simulink model "LQI_control"  (R2020a)
settings: Solver=ode4  StartTime=0.0  StopTime=t  FixedStep=0.01  RelTol=1e-3
values from neighbouring files (symbols this model uses):
  A = [-0.0226 -36.6 -18.9 -32.1 ;            0 -1.9  0.983     0;       0.0123 -11.7 -2.63     0;            0     0     1     0]    [Sylvester.m]
  B = [0      0;      -0.414 0;      -77.8 22.4;      0     0]    [Sylvester.m]
  C = [0  57.3  0  0;      0    0   0  57.3]    [Sylvester.m]
  D = zeros(2,2)    [Sylvester.m]
  K = lqi(sys,Q,R)    [Sylvester.m]
  L = ones(4,2)    [Sylvester.m]
  M = eye(4)*diag([-6 -5 -7 -8])    [Sylvester.m]
  N = double(nT*B-L*D)    [Sylvester.m]
  nT = double([cT(1) cT(2) cT(3) cT(4);       cT(5) cT(6) cT(7) cT(8);       cT(9) cT(10) cT(11) cT(12);       cT(13) cT(14) cT(15) cT(16)])    [Sylvester.m]
undefined symbols (not defined in the file or in its folder): sigbuilder_block, x0, z0
settings Model: Creator=grzyb  LastModifiedBy=grzyb

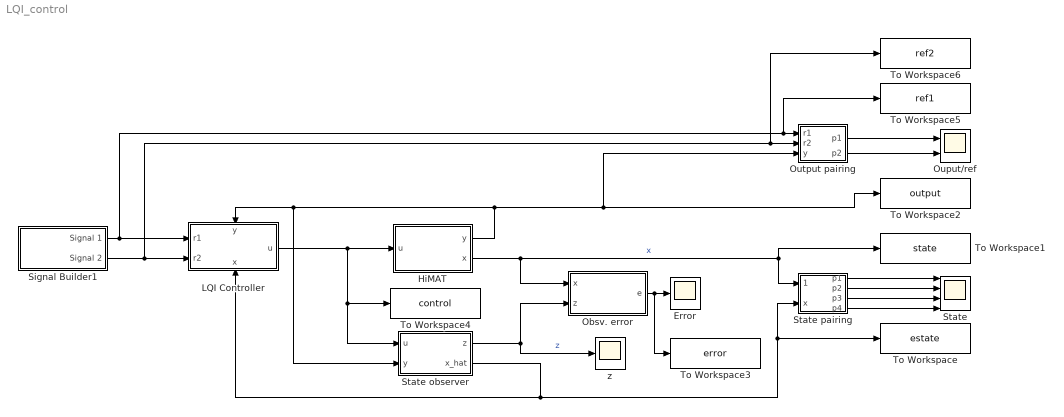
== system LQI_control ==
  Error : Scope
  HiMAT : Subsystem
  LQI Controller : Subsystem
      settings: PortSchema="{\"entries\":[{\"content\":{\"sides\":[{\"content\":{\"connectorIds\":[\"In1\",\"In2\"]},\"type\":\"ConnectorPlacement.EquallySpacedRectSide\",\"uuid\":\"e3c02560-f56c-4735-be79-63117d7509a6\"},{\"content\":{\"connectorIds\":[\"Out1\"],\"side\":\"RIGHT\"},\"type\":\"ConnectorPlacement.EquallySpacedRectSide\",\"uuid\":\"a1606b3d-8e51-4c6c-b27f-ff2fba47f691\"},{\"content\":{\"connectorIds\":[\"In3\"],\"side\":\"TOP\"},\"type\":\"ConnectorPlacement.EquallySpacedRectSide\",\"uuid\":\"974286de-bdd3-4a89-9cf9-bd41fa972893\"},{\"content\":{\"connectorIds\":[\"In4\"],\"side\":\"BOTTOM\"},\"type\":\"ConnectorPlacement.EquallySpacedRectSide\",\"uuid\":\"2d098620-1fb3-495b-92dc-71a09978788a\"}]},\"type\":\"ConnectorPlacement.EquallySpacedConnector\",\"uuid\":\"f97bae00-d8a8-4485-bbc3-7ca32c22b62e\"}],\"packageUris\":[\"http://schema.mathworks.com/mf0/Connector/19700101\"],\"version\":\"1.0\"}"
  Obsv. error : Subsystem
  Ouput/ref : Scope  NumInputPorts=2
  Output pairing : Subsystem
  Signal Builder1 : Subsystem  Tag=STV Subsys  LoadFcn=sigbuilder_block('load');  StartFcn=sigbuilder_block('start');  StopFcn=sigbuilder_block('stop');  ClipboardFcn=sigbuilder_block('clipboard');  mask(Sigbuilder block){tuvar=[0:10]}
      mask help: Simulink:masks:SigbuilderBlock_MD
      mask init:
      | if ~strcmp(get_param(bdroot(gcbh),'SimulationStatus'),'stopped') tuvar = sigbuilder_block('maskInit'); end
      settings: CopyFcn=sigbuilder_block('copy');  DeleteFcn=sigbuilder_block('delete');  ModelCloseFcn=sigbuilder_block('modelClose');  PreSaveFcn=sigbuilder_block('preSave');  PauseFcn=sigbuilder_block('pause');  ContinueFcn=sigbuilder_block('continue');  NameChangeFcn=sigbuilder_block('namechange');  OpenFcn=sigbuilder_block('open',[437.6 199.2 550.4 400 ]);  CloseFcn=sigbuilder_block('close');
      mask Display: plot(0, 0, 100, 100,[2, 2, 32, 32, 2], [68, 8, 8, 68, 68],[32, 2], [38, 38], [32, 19, 2],[53, 60, 44], [32, 17, 17, 2],[16, 16, 31, 31]);txt = getActiveGroup(gcbh);text(2, 100, txt,'verticalAlignment', 'top');
  State : Scope  NumInputPorts=4
  State observer : Subsystem
  State pairing : Subsystem
  To Workspace : ToWorkspace  VariableName=estate  SaveFormat=Structure  SampleTime=-1
  To Workspace1 : ToWorkspace  VariableName=state  SaveFormat=Structure  SampleTime=-1
  To Workspace2 : ToWorkspace  VariableName=output  SaveFormat=Structure  SampleTime=-1
  To Workspace3 : ToWorkspace  VariableName=error  SaveFormat=Structure  SampleTime=-1
  To Workspace4 : ToWorkspace  VariableName=control  SaveFormat=Structure  SampleTime=-1
  To Workspace5 : ToWorkspace  VariableName=ref1  SaveFormat=Structure  SampleTime=-1
  To Workspace6 : ToWorkspace  VariableName=ref2  SaveFormat=Structure  SampleTime=-1
  z : Scope
  wires:
  State pairing/1(p1) -> State/1
  State pairing/2(p2) -> State/2
  State pairing/3(p3) -> State/3
  State pairing/4(p4) -> State/4
  LQI Controller/1(u) -> To Workspace4/1, State observer/1(u), HiMAT/1(u)
  HiMAT/2(x) -> To Workspace1/1, State pairing/1(x_hat), Obsv. error/1(x)  "x"
  State observer/1(z) -> z/1, Obsv. error/2(z)  "z"
  State observer/2(x_hat) -> LQI Controller/4(x), To Workspace/1, State pairing/2(x)
  HiMAT/1(y) -> Output pairing/3(y), To Workspace2/1, State observer/2(y), LQI Controller/3(y)
  Obsv. error/1(e) -> To Workspace3/1, Error/1
  Output pairing/1(p1) -> Ouput/ref/1
  Output pairing/2(p2) -> Ouput/ref/2
  Signal Builder1/1(Signal 1) -> To Workspace5/1, Output pairing/1(r1), LQI Controller/1(r1)
  Signal Builder1/2(Signal 2) -> To Workspace6/1, Output pairing/2(r2), LQI Controller/2(r2)

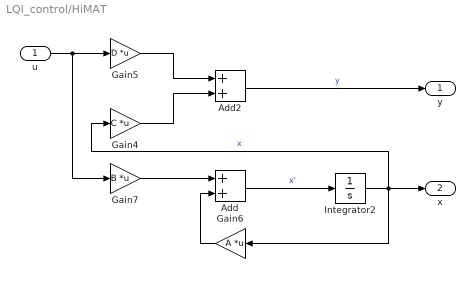
== system LQI_control/HiMAT ==
  u : Inport
  Add : Sum
  Add2 : Sum
  Gain4 : Gain  Gain=C  Multiplication=Matrix(K*u)
  Gain5 : Gain  Gain=D  Multiplication=Matrix(K*u)
  Gain6 : Gain  Gain=A  Multiplication=Matrix(K*u)
  Gain7 : Gain  Gain=B  Multiplication=Matrix(K*u)
  Integrator2 : Integrator  InitialCondition=x0
  y : Outport
  x : Outport  Port=2
  wires:
  Gain5/1 -> Add2/1
  Gain6/1 -> Add/2
  u/1 -> Gain7/1, Gain5/1
  Gain4/1 -> Add2/2
  Add/1 -> Integrator2/1  "x'"
  Add2/1 -> y/1  "y"
  Gain7/1 -> Add/1
  Integrator2/1 -> Gain4/1, Gain6/1, x/1  "x"

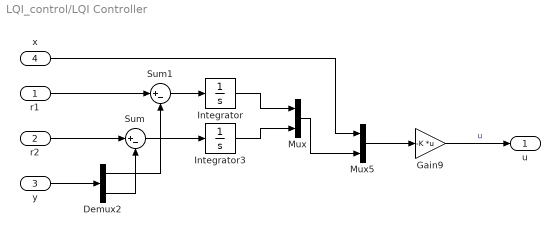
== system LQI_control/LQI Controller ==
  r1 : Inport
  r2 : Inport  Port=2
  y : Inport  Port=3
  x : Inport  Port=4
  Demux2 : Demux  Outputs=2
  Gain9 : Gain  Gain=-K  Multiplication=Matrix(K*u)
  Integrator : Integrator
  Integrator3 : Integrator
  Mux : Mux  Inputs=2
  Mux5 : Mux  Inputs=2
  Sum : Sum  Inputs=|+-
  Sum1 : Sum  Inputs=|+-
  u : Outport
  wires:
  y/1 -> Demux2/1
  Sum1/1 -> Integrator/1
  Integrator3/1 -> Mux/2
  Sum/1 -> Integrator3/1
  Integrator/1 -> Mux/1
  Demux2/2 -> Sum/2
  r2/1 -> Sum/1
  Mux5/1 -> Gain9/1
  x/1 -> Mux5/1
  Mux/1 -> Mux5/2
  Demux2/1 -> Sum1/2
  Gain9/1 -> u/1  "u"
  r1/1 -> Sum1/1

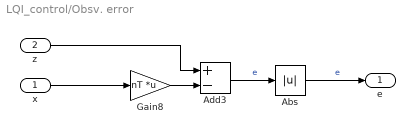
== system LQI_control/Obsv. error ==
  x : Inport
  z : Inport  Port=2
  Abs : Abs
  Add3 : Sum  Inputs=+-
  Gain8 : Gain  Gain=nT  Multiplication=Matrix(K*u)
  e : Outport
  wires:
  z/1 -> Add3/1
  x/1 -> Gain8/1
  Gain8/1 -> Add3/2
  Add3/1 -> Abs/1  "e"
  Abs/1 -> e/1  "e"

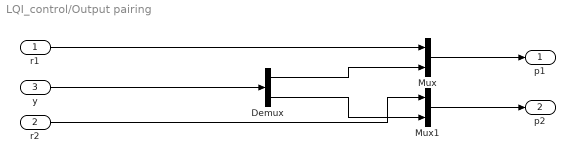
== system LQI_control/Output pairing ==
  r1 : Inport
  r2 : Inport  Port=2
  y : Inport  Port=3
  Demux : Demux  Outputs=2
  Mux : Mux  Inputs=2
  Mux1 : Mux  Inputs=2
  p1 : Outport
  p2 : Outport  Port=2
  wires:
  r1/1 -> Mux/1
  Mux/1 -> p1/1
  Demux/2 -> Mux1/2
  Demux/1 -> Mux/2
  Mux1/1 -> p2/1
  y/1 -> Demux/1
  r2/1 -> Mux1/1

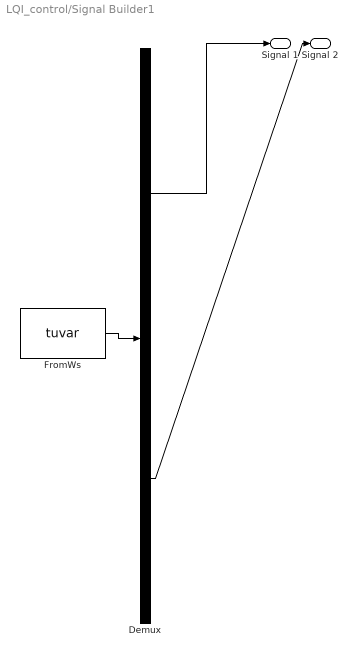
== system LQI_control/Signal Builder1 ==
  Demux : Demux  Tag=STV Demux  Outputs=2
      settings: DisplayOption=none
  FromWs : FromWorkspace  Tag=STV FromWs  VariableName=tuvar
      SigBuilderData=|
      | common.afterFinalStr = 'Extrapolate'
      | common.sampleTime = 0
      | dataSet.timeRange = [0 50]
      | dataSet.name = 'Group 1'
      | sbobj.Groups.Name = 'Group 1'
      | sbobj.Groups.Signals(1).Name = 'Signal 1'
      | sbobj.Groups.Signals(1).XData = [0 25 25 50]
      | sbobj.Groups.Signals(1).YData = [0 0 -5 -5]
      | sbobj.Groups.Signals(2).Name = 'Signal 2'
      | sbobj.Groups.Signals(2).XData = [0 10 10 50]
      | sbobj.Groups.Signals(2).YData = [0 0 2 2]
      | sbobj.Groups.TimeRange = [0 50]
  Signal 1 : Outport  Tag=STV Outport
  Signal 2 : Outport  Tag=STV Outport  Port=2
  wires:
  FromWs/1 -> Demux/1
  Demux/1 -> Signal 1/1
  Demux/2 -> Signal 2/1

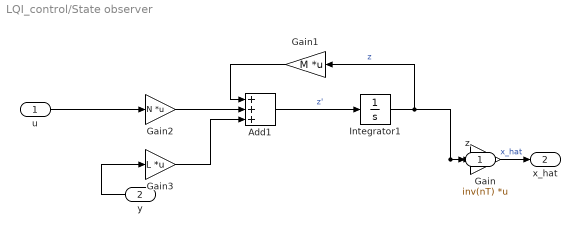
== system LQI_control/State observer ==
  u : Inport
  y : Inport  Port=2
  Add1 : Sum  Inputs=+++
  Gain : Gain  Gain=inv(nT)  Multiplication=Matrix(K*u)
  Gain1 : Gain  Gain=M  Multiplication=Matrix(K*u)
  Gain2 : Gain  Gain=N  Multiplication=Matrix(K*u)
  Gain3 : Gain  Gain=L  Multiplication=Matrix(K*u)
  Integrator1 : Integrator  InitialCondition=z0
  z : Outport
  x_hat : Outport  Port=2
  wires:
  Add1/1 -> Integrator1/1  "z'"
  Gain1/1 -> Add1/1
  Gain/1 -> x_hat/1  "x_hat"
  u/1 -> Gain2/1
  Integrator1/1 -> Gain/1, z/1, Gain1/1  "z"
  y/1 -> Gain3/1
  Gain2/1 -> Add1/2
  Gain3/1 -> Add1/3

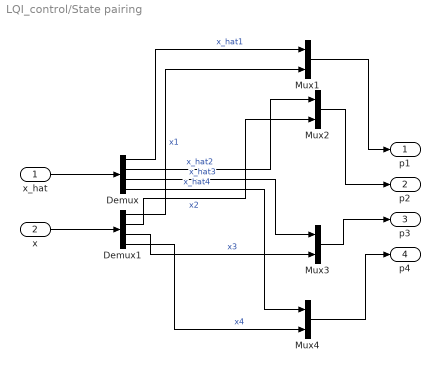
== system LQI_control/State pairing ==
  x_hat : Inport
  x : Inport  Port=2
  Demux : Demux
  Demux1 : Demux
  Mux{1..4} (4 alike) : Mux  Inputs=2
  p1 : Outport
  p2 : Outport  Port=2
  p3 : Outport  Port=3
  p4 : Outport  Port=4
  wires:
  Demux/2 -> Mux2/1  "x_hat2"
  Demux/4 -> Mux4/1  "x_hat4"
  Demux1/4 -> Mux4/2  "x4"
  Demux1/1 -> Mux1/2  "x1"
  Demux/1 -> Mux1/1  "x_hat1"
  Mux1/1 -> p1/1
  Demux/3 -> Mux3/1  "x_hat3"
  Mux2/1 -> p2/1
  Demux1/3 -> Mux3/2  "x3"
  Mux4/1 -> p4/1
  Demux1/2 -> Mux2/2  "x2"
  x/1 -> Demux1/1
  x_hat/1 -> Demux/1
  Mux3/1 -> p3/1
